simulink model "Monopolar_SPWM"  (R2023a)
settings: Solver=VariableStepAuto  StartTime=0.0  StopTime=0.2  RelTol=1e-3
libraries: spsIGBTDiodeLib x4, spsCurrentMeasurementLib x1, spsDCVoltageSourceLib x1, spsRMSLib x1, spsSeriesRLCBranchLib x1, spsTHDLib x1, spsTriangleGeneratorLib x1, spsVoltageMeasurementLib x1, sps_lib x1
settings Model: Creator=Rizwan computers  LastModifiedBy=Rizwan computers
settings DataIOCC: ReturnWorkspaceOutputs=off

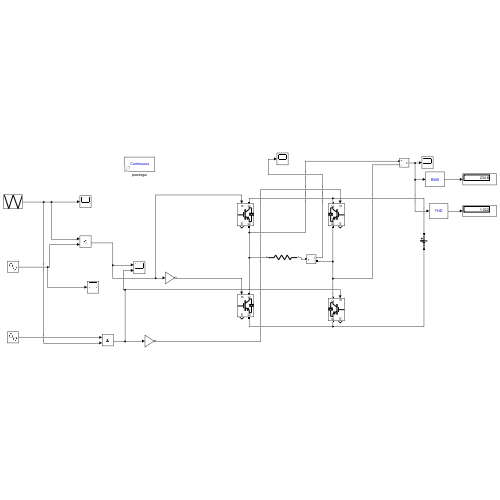
[thumbnail: Simulink's stored preview of the top-level diagram]
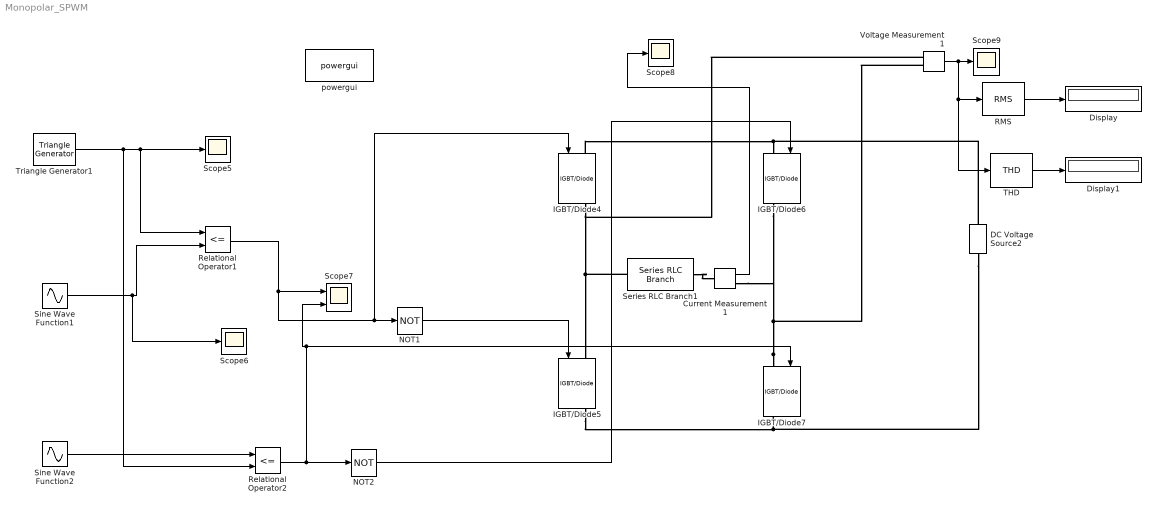
== system Monopolar_SPWM ==
  Current Measurement1 : spsCurrentMeasurementLib/Current Measurement  PhasorSimulation=off  OutputType=Complex  PSBequivalent=0
  DC Voltage Source2 : spsDCVoltageSourceLib/DC Voltage Source  Amplitude=350  Measurements=None
  Display : Display
  Display1 : Display
  IGBT/Diode{4..7} (4 alike) : spsIGBTDiodeLib/IGBT//Diode  Ron=1e-3  Rs=1e5  Cs=inf  Measurements=on
  NOT1 : Logic  Operator=NOT  IconShape=distinctive  AllPortsSameDT=off  OutDataTypeStr=boolean
  NOT2 : Logic  Operator=NOT  IconShape=distinctive  AllPortsSameDT=off  OutDataTypeStr=boolean
  RMS : spsRMSLib/RMS  TrueRMS=on  Freq=60  RMSInit=120  Ts=0
  Relational Operator1 : RelationalOperator  Operator=<=  OutDataTypeStr=boolean  RndMeth=Simplest  InputSameDT=off
  Relational Operator2 : RelationalOperator  Operator=<=  OutDataTypeStr=boolean  RndMeth=Simplest  InputSameDT=off
  Scope{5..6,8..9} (4 alike) : Scope
  Scope7 : Scope  NumInputPorts=2
  Series RLC Branch1 : spsSeriesRLCBranchLib/Series RLC Branch  LConnTagsString=__new0  RConnTagsString=__new0  BranchType=R  Resistance=100  Inductance=1e-3  SetiL0=off  InitialCurrent=0  Capacitance=1e-6  Setx0=off  InitialVoltage=0  Measurements=None
  Sine Wave Function1 : Sin  Amplitude=0.4  Frequency=314  SampleTime=0
  Sine Wave Function2 : Sin  Amplitude=0.9  Frequency=314.2  Phase=pi*.9  SampleTime=0
  THD : spsTHDLib/THD  Freq=60  Ts=0
  Triangle Generator1 : spsTriangleGeneratorLib/Triangle Generator  Freq=5e3  Phase=180  Ts=0
  Voltage Measurement1 : spsVoltageMeasurementLib/Voltage Measurement  PhasorSimulation=off  OutputType=Complex  PSBequivalent=0
  powergui : sps_lib/powergui  Priority=1  SimulationMode=Continuous  SampleTime=50e-6  frequency=60  Iterations=50  frequencyindice=0  Pbase=100e6  ErrMax=1e-4  UnitsV=kV  UnitsW=MW  buscounter=0  FunctionMessages=off  echomessages=off  EnableUseOfTLC=off  CurrentSourceSwitches=off  DisableSnubberDevices=off  DisableRonSwitches=off  DisableVfSwitches=off  DisplayEquations=off  AutomaticDiscreteSolvers=off  SolverType=Tustin/Backward Euler (TBE)  Interpol=off  ExternalGateDelay=off  methode=off  Ts=100  x0status=blocks  SPID=on  SwTol=0  HookPort=off  NonlinearTolerance=1e-4  nMaxIteration=100  ContinueOnMaxIteration=off  RestoreLinks=warning  ResistiveCurrentMeasurement=off  Frange=[0:2:500]  Ylog=off  Xlog=on  ShowGrid=off  save=off  variable=ZData  structure=0  ZoomFFT=off  StartTime=0.0  cycles=1  DisplayStyle=1  fundamental=60  FreqAxis=off  MaxFrequency=1000  frequencyindicesteady=1  RmsSteady=1  display=off
  wires:
  THD/1 -> Display1/1
  Triangle Generator1/1 -> Relational Operator2/2, Relational Operator1/1, Scope5/1
  NOT2/1 -> IGBT/Diode6/1
  Relational Operator1/1 -> Scope7/1, IGBT/Diode4/1, NOT1/1
  Sine Wave Function2/1 -> Relational Operator2/1
  NOT1/1 -> IGBT/Diode5/1
  Sine Wave Function1/1 -> Relational Operator1/2, Scope6/1
  Relational Operator2/1 -> Scope7/2, IGBT/Diode7/1, NOT2/1
  Current Measurement1/1 -> Scope8/1
  RMS/1 -> Display/1
  Voltage Measurement1/1 -> THD/1, RMS/1, Scope9/1
  connections:
  DC Voltage Source2/RConn1 -- IGBT/Diode6/LConn1 -- IGBT/Diode4/LConn1
  Series RLC Branch1/LConn1 -- IGBT/Diode5/LConn1 -- Voltage Measurement1/LConn1 -- IGBT/Diode4/RConn1
  IGBT/Diode7/RConn1 -- IGBT/Diode5/RConn1 -- DC Voltage Source2/LConn1
  IGBT/Diode7/LConn1 -- IGBT/Diode6/RConn1 -- Current Measurement1/RConn1 -- Voltage Measurement1/LConn2
  Series RLC Branch1/RConn1 -- Current Measurement1/LConn1
